simulink model "BlinkerCAN"  (R2017b)
settings: Solver=FixedStepAuto  StartTime=0.0  StopTime=10.0  RelTol=1e-3
PreLoadFcn:
  | waijung.modelPreload; % Required for working with Waijung Blockset. Do not remove.
undefined symbols (not defined in the file): HSEOSC, Link, LQFP100, ST, STM32F407VG
libraries: simulink x22, hdlsllib x17, stm32f4_canbus_lib x5, stm32f4_io_lib x1, stm32f4_device_config_lib x1
CloseFcn:
  | waijung.modelClose; % Required for working with Waijung Blockset. Do not remove.
settings Model: Creator=labuser  LastModifiedBy=labuser
settings OptimizationCC: DefaultParameterBehavior=Inlined  PassReuseOutputArgsAs=Individual arguments
settings DebuggingCC: ParameterTunabilityLossMsg=error
settings HardwareCC: ProdBitPerPointer=32  ProdBitPerSizeT=32  ProdBitPerPtrDiffT=32  ProdLargestAtomicFloat=None  ProdIntDivRoundTo=Undefined  ProdWordSize=32  ProdHWDeviceType=ARM Compatible->Cortex - M4  TargetEndianess=LittleEndian  TargetHWDeviceType=ARM Compatible->Cortex - M4
settings SFSimCC: MATLABDynamicMemAlloc=off
settings RTWCC: SystemTargetFile=stm32f4.tlc  GenerateMakefile=off  TemplateMakefile=ert_default_tmf  Description=STM32F4 Target  GenerateReport=on  IncludeHyperlinkInReport=on  LaunchReport=on  GenerateTraceInfo=on  GenerateTraceReport=on  GenerateTraceReportSl=on  GenerateTraceReportSf=on  GenerateTraceReportEml=on
settings CodeAppCC: ForceParamTrailComments=on  IgnoreCustomStorageClasses=off  OperatorAnnotations=on  SimulinkDataObjDesc=on  SFDataObjDesc=on  InsertBlockDesc=on
settings STFCustomTargetCC: TargetLangStandard=C99 (ISO)  MultiwordLength=256  ModelReferenceCompliant=off  CombineOutputUpdateFcns=on  ERTCustomFileBanners=on  SupportContinuousTime=off  SupportNonInlinedSFcns=off  RemoveResetFunc=on  MATLABClassNameForMDSCustomization=Simulink.SoftwareTarget.ERTCustomization  GRTInterface=off  SystemTargetFile=stm32f4.tlc
settings ERTTargetCC: TargetLangStandard=C99 (ISO)  ModelReferenceCompliant=off  ParMdlRefBuildCompliant=off  CompOptLevelCompliant=off  ConcurrentExecutionCompliant=off  ModelStepFunctionPrototypeControlCompliant=off  CPPClassGenCompliant=off  UseToolchainInfoCompliant=off  InlinedParameterPlacement=NonHierarchical  ERTSrcFileBannerTemplate=stm32f4_code_template.cgt  ERTHdrFileBannerTemplate=stm32f4_code_template.cgt  ERTDataSrcFileTemplate=stm32f4_code_template.cgt  ERTDataHdrFileTemplate=stm32f4_code_template.cgt  ERTCustomFileTemplate=stm32f4_file_process.tlc

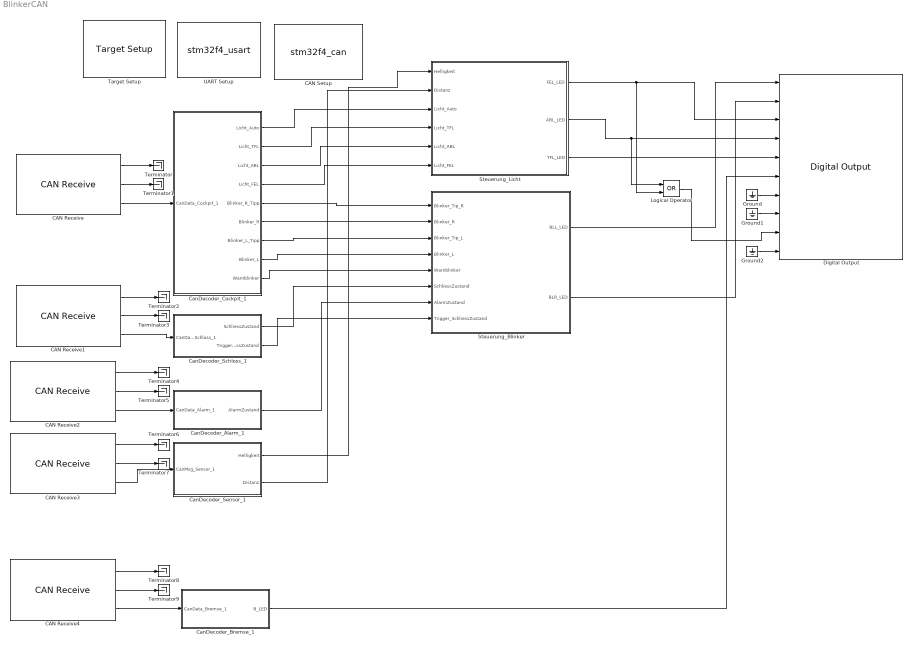
== system BlinkerCAN ==
  CAN Receive : stm32f4_canbus_lib/CAN Receive  conf=Rx  canmodule=1  idtype=Standard  filtertype=Specific  id=14  idmask=00000000  enableisr=off  usedlc=off  datatype=single  data0type=uint8  data1type=Not used  data2type=Not used  data3type=Not used  data4type=Not used  data5type=Not used  data6type=Not used  data7type=Not used  buffersize=8  sampletime=-1  sampletimestr=-1  blockid=CANReceive  inputarray=[]  inputlabelarray={}  outputarray=[ 5, 7, 3]  outputlabelarray={ 'Msg Pending','ID', 'D0 (uint8)' }  compat=0  confstr="[\"Standard\",\"Specific\",\"14\",\"0\",\"off\",\"uint8\",\"Not used\",\"Not used\",\"Not used\",\"Not used\",\"Not used\",\"Not used\",\"Not used\",\"8\",\"1C0\",\"0\",\"FFE0\",\"4\"]"
  CAN Receive1 : stm32f4_canbus_lib/CAN Receive  conf=Rx  canmodule=1  idtype=Standard  filtertype=Specific  id=25  idmask=00000000  enableisr=off  usedlc=off  datatype=single  data0type=uint8  data1type=Not used  data2type=Not used  data3type=Not used  data4type=Not used  data5type=Not used  data6type=Not used  data7type=Not used  buffersize=8  sampletime=-1  sampletimestr=-1  blockid=CANReceive1  inputarray=[]  inputlabelarray={}  outputarray=[ 5, 7, 3]  outputlabelarray={ 'Msg Pending','ID', 'D0 (uint8)' }  compat=0  confstr="[\"Standard\",\"Specific\",\"25\",\"0\",\"off\",\"uint8\",\"Not used\",\"Not used\",\"Not used\",\"Not used\",\"Not used\",\"Not used\",\"Not used\",\"8\",\"320\",\"0\",\"FFE0\",\"4\"]"
  CAN Receive2 : stm32f4_canbus_lib/CAN Receive  conf=Rx  canmodule=1  idtype=Standard  filtertype=Specific  id=24  idmask=00000000  enableisr=off  usedlc=off  datatype=single  data0type=uint8  data1type=Not used  data2type=Not used  data3type=Not used  data4type=Not used  data5type=Not used  data6type=Not used  data7type=Not used  buffersize=8  sampletime=-1  sampletimestr=-1  blockid=CANReceive2  inputarray=[]  inputlabelarray={}  outputarray=[ 5, 7, 3]  outputlabelarray={ 'Msg Pending','ID', 'D0 (uint8)' }  compat=0  confstr="[\"Standard\",\"Specific\",\"24\",\"0\",\"off\",\"uint8\",\"Not used\",\"Not used\",\"Not used\",\"Not used\",\"Not used\",\"Not used\",\"Not used\",\"8\",\"300\",\"0\",\"FFE0\",\"4\"]"
  CAN Receive3 : stm32f4_canbus_lib/CAN Receive  conf=Rx  canmodule=1  idtype=Standard  filtertype=Specific  id=32  idmask=00000000  enableisr=off  usedlc=off  datatype=single  data0type=uint16  data1type=Not used  data2type=Not used  data3type=Not used  data4type=Not used  data5type=Not used  data6type=Not used  data7type=Not used  buffersize=8  sampletime=-1  sampletimestr=-1  blockid=CANReceive3  inputarray=[]  inputlabelarray={}  outputarray=[ 5, 7, 5]  outputlabelarray={ 'Msg Pending','ID', 'D0 (uint16)' }  compat=0  confstr="[\"Standard\",\"Specific\",\"32\",\"0\",\"off\",\"uint16\",\"Not used\",\"Not used\",\"Not used\",\"Not used\",\"Not used\",\"Not used\",\"Not used\",\"8\",\"400\",\"0\",\"FFE0\",\"4\"]"
  CAN Receive4 : stm32f4_canbus_lib/CAN Receive  conf=Rx  canmodule=1  idtype=Standard  filtertype=Specific  id=10  idmask=00000000  enableisr=off  usedlc=off  datatype=single  data0type=uint8  data1type=Not used  data2type=Not used  data3type=Not used  data4type=Not used  data5type=Not used  data6type=Not used  data7type=Not used  buffersize=8  sampletime=-1  sampletimestr=-1  blockid=CANReceive4  inputarray=[]  inputlabelarray={}  outputarray=[ 5, 7, 3]  outputlabelarray={ 'Msg Pending','ID', 'D0 (uint8)' }  compat=0  confstr="[\"Standard\",\"Specific\",\"10\",\"0\",\"off\",\"uint8\",\"Not used\",\"Not used\",\"Not used\",\"Not used\",\"Not used\",\"Not used\",\"Not used\",\"8\",\"140\",\"0\",\"FFE0\",\"4\"]"
  CAN Setup : S-Function  FunctionName=stm32f4_can  Parameters=conf,canmodule,0,inputarray,outputarray,'','',confstr,sampletime,sampletimestr,blockid  SFunctionDeploymentMode=off  EnableBusSupport=off  mask(stm32f4_can){conf=Setup, canmodule=1, advance=off, bitrate_select=125000, sjw=1tq, bs1=14tq, bs2=6tq, timingconf=Prescaler, brp=16, bitrate=125000, tq=3.8095e-07, autoretransmission=Disable, remaptxpin=D1, remaprxpin=D0, sampletime=-1, sampletimestr=-1, blockid=CANSetup, inputarray=[], inputlabelarray={}, outputarray=[], outputlabelarray={}, compat=0, confstr=["125000","16","D","1","D","0","1tq","14tq","6tq","ENABLE"], presc=16, txportstr=D, txpinstr=1, rxportstr=D, rxpinstr=0, lastmodule=1}
      mask prompts: conf "Configuration"; canmodule "CAN Module"; advance "Advance configuration"; bitrate_select "Baud rate (bps)"; sjw "Resync Jump Width (SJW)"; bs1 "Bit segment 1 (BS1) + PROP_SEG"; bs2 "Bit segment 2 (BS2)"; timingconf "Adjust"; brp "Baud rate prescaler (BRP)"; bitrate "Baud rate (bps)"; tq "Time Quantum (Second), tq"; autoretransmission "Auto Re-transmission"; remaptxpin "CAN Tx pin"; remaprxpin "CAN Rx pin"; sampletime "Sample time (sec)"; sampletimestr "Compiled sample time (sec) in string"; inputarray "Input port"; inputlabelarray "Input port label"; outputarray "Output port"; outputlabelarray "Output port label"; compat "Compatibility (Reserved for future use)"; confstr "Configuration String"; presc "Prescale"; txportstr "Tx port string"; txpinstr "Tx pin string"; rxportstr "Rx port string"; rxpinstr "Rx pin string"; lastmodule "Last module selected"
      mask help:
      | This block setups CAN Module.
      |
      | Auto Re-transmission,
      |  - Enable: The CAN hardware will automatically retransmit the message until it has been
      | successfully transmitted according to the CAN standard.
      |  - Disable: A message will be transmitted only once, independently of the transmission result
      | (successful, error or arbitration lost).
      mask init:
      | stm32f4_can_callback('init');
      mask Help: web(fullfile(waijungdocroot,'stm32f4_can_setup.htm'), '-browser')
      mask TypeOptions conf: Setup
      mask TypeOptions canmodule: 1 | 2
      mask Callback canmodule: stm32f4_can_callback('canmodule');
      mask Callback advance: stm32f4_can_callback('advance');
      mask TypeOptions bitrate_select: 125000 | 250000 | 500000 | 1000000
      mask Callback bitrate_select: stm32f4_can_callback('bitrate_select');
      mask TypeOptions sjw: 1tq | 2tq | 3tq | 4tq
      mask TypeOptions bs1: 1tq | 2tq | 3tq | 4tq | 5tq | 6tq | 7tq | 8tq | 9tq | 10tq | 11tq | 12tq | 13tq | 14tq | 15tq | 16tq
      mask Callback bs1: stm32f4_can_callback('timingconf');
      mask TypeOptions bs2: 1tq | 2tq | 3tq | 4tq | 5tq | 6tq | 7tq | 8tq
      mask Callback bs2: stm32f4_can_callback('timingconf');
      mask TypeOptions timingconf: Prescaler | Baudrate
      mask Callback timingconf: stm32f4_can_callback('timingconf');
      mask Callback brp: stm32f4_can_callback('timingconf');
      mask Callback bitrate: stm32f4_can_callback('timingconf');
      mask TypeOptions autoretransmission: Enable | Disable
      mask TypeOptions remaptxpin: Not used | A12 | B9 | D1
      mask Callback remaptxpin: stm32f4_can_callback('remaptxpin');
      mask TypeOptions remaprxpin: Not used | A11 | B8 | D0
      mask Callback remaprxpin: stm32f4_can_callback('remaprxpin');
      mask Callback sampletime: stm32f4_can_callback('sampletime');
      mask Callback sampletimestr: stm32f4_can_callback('sampletimestr');
      mask Callback blockid: stm32f4_can_callback('blockid');
      mask Display: text(0.5, 0.5, 'CAN1_Setup\nSpeed (bps): 125000\nTx/Rx pin: D1/D0','ver','middle','hor','center');
  CanDecoder_Alarm_1 : Subsystem
  CanDecoder_Bremse_1 : Subsystem
  CanDecoder_Cockpit_1 : Subsystem
  CanDecoder_Schloss_1 : Subsystem
  CanDecoder_Sensor_1 : Subsystem
  Digital Output : stm32f4_io_lib/Digital Output  use_bitband=on  port=C  speed=100  porttype=Push Pull  porttypestr=PP  use_pin0=on  use_pin1=on  use_pin2=on  use_pin3=on  use_pin4=on  use_pin5=on  use_pin6=on  use_pin7=on  use_pin8=on  use_pin9=on  use_pin10=off  use_pin11=off  use_pin12=off  use_pin13=off  use_pin14=off  use_pin15=off  pinstr=GPIO_Pin_0 | GPIO_Pin_1 | GPIO_Pin_2 | GPIO_Pin_3 | GPIO_Pin_4 | GPIO_Pin_5 | GPIO_Pin_6 | GPIO_Pin_7 | GPIO_Pin_8 | GPIO_Pin_9  usedpinarray="[1  1  1  1  1  1  1  1  1  1  0  0  0  0  0  0]"  bitbandingstr=|  sampletime=-1  sampletimestr=-1  blockid=DigitalOutput  enablecustomportlabel=off  globalinit=off  cinputportlabel=In1, In2  coutputportlabel=0
      | #define DigitalOutput_C0 Peripheral_BB(GPIOC->ODR, 0)  /* Output pin */
      | #define DigitalOutput_C1 Peripheral_BB(GPIOC->ODR, 1)  /* Output pin */
      | #define DigitalOutput_C2 Peripheral_BB(GPIOC->ODR, 2)  /* Output pin */
      | #define DigitalOutput_C3 Peripheral_BB(GPIOC->ODR, 3)  /* Output pin */
      | #define DigitalOutput_C4 Peripheral_BB(GPIOC->ODR, 4)  /* Output pin */
      | #define DigitalOutput_C5 Peripheral_BB(GPIOC->ODR, 5)  /* Output pin */
      | #define DigitalOutput_C6 Peripheral_BB(GPIOC->ODR, 6)  /* Output pin */
      | #define DigitalOutput_C7 Peripheral_BB(GPIOC->ODR, 7)  /* Output pin */
      | #define DigitalOutput_C8 Peripheral_BB(GPIOC->ODR, 8)  /* Output pin */
      | #define DigitalOutput_C9 Peripheral_BB(GPIOC->ODR, 9)  /* Output pin */
      settings: SourceProductName=Waijung Blockset
  Ground : Ground
  Ground1 : Ground
  Ground2 : Ground
  Logical Operator : Logic  Operator=OR  AllPortsSameDT=off  OutDataTypeStr=boolean
  Steuerung_Blinker : Stateflow chart  TreatAsAtomicUnit=on
  Steuerung_Licht : Stateflow chart  TreatAsAtomicUnit=on
  Target Setup : stm32f4_device_config_lib/Target Setup  Priority=100  compiler=GNU ARM  previous_compiler=GNU ARM  mcu=STM32F407VG (LQFP100)  mcustr=STM32F407VG  clockconfig=HSEOSC-8MHz  system_stm32f4xx_c_path=C:\Users\labuser\Desktop\waijung17_03a\targets\stm32f4_target\stm32f4\utils\system_stm32f4xx_default\STM32F40_41xxx\hseosc8mhz  showmemoryconfiguration=off  stacksize=0x2000  heapsize=0x2000  enableautocompiledownload=on  fullchiperase=off  programmerinterface=ST-Link  editctrlstr=on  compilercontrolstr=$(patsubst %, -I%, .) -mcpu=cortex-m4 -mthumb -mthumb-interwork -mfloat-abi=hard -mfpu=fpv4-sp-d16 -ffast-math -Wall -Wextra -Ofast  assemblercontrolstr=$(patsubst %, -I%, .) -mcpu=cortex-m4 -mthumb -mthumb-interwork -mfloat-abi=hard -mfpu=fpv4-sp-d16 -ffast-math -Wall -Wextra -Ofast -Wa,-amhls=$(<:.s=.lst) -D__STACK_SIZE=$(STACK_SIZE) -D__HEAP_SIZE=$(HEAP_SIZE)  linkercontrolstr=-T$(LD_SCRIPT) -g -Wl,-Map=$(MAP),--cref,--no-warn-mismatch -mcpu=cortex-m4 -mthumb -mthumb-interwork -mfloat-abi=hard -mfpu=fpv4-sp-d16 -specs=nosys.specs  runafterdownload=on  execprofile=None  profileruart=3  profilerbaud=500000  profilertxpin=D8  profilerinitstr=0.01,168000000,1680000,500000,0  manualsetsampletime=off  sampletime=0.01  blockid=TargetSetup  systickreloadvalue=1680000  hseval=8000000  lastprofileruart=3  hclk=168000000  flashorigin=0x8000000  flashlength=1024k  ramorigin=0x20000000  ramlength=128k  useextram=off
      settings: SourceProductName=Waijung Blockset
  Terminator{,1..9} (10 alike) : Terminator
  UART Setup : S-Function  Priority=1  FunctionName=stm32f4_usart  Parameters=configuration,uartmodule,transfer,baudrate,inputtype,outputtype,confstr,binheaderarray,binterminatorarray,asciiheader,asciiterminator,bindatalength,packetmode,varname,sampletime,sampletimestr,blockid  SFunctionDeploymentMode=off  EnableBusSupport=off  mask(stm32f4_usart){configuration=Setup, uartmodule=2, baudrate=115200, databits=8, parity=No, stopbit=1, remaptxpin=A2, remaprxpin=A3, flowcontrol=None, remapctspin=Not used, remaprtspin=Not used, advanceoptions=off, rxbuffersize=512, txbuffersize=512, transfer=Blocking, packetmode=Ascii, binheader='7E 7E', binterminator='03 03', porttype_double=1, porttype_single=0, porttype_int8=1, porttype_uint8=0, porttype_int16=0, porttype_uint16=0, porttype_int32=0, porttype_uint32=0, asciiformat='%d,%f', rx_asciiterminator=CRLF (0x0D 0x0A - "\r\n"), tx_asciiterminator=CR (0x0D - "\r"), storagename=<empty>, varname=, inputtype=[0], outputtype=[0], binheaderarray=[0], binterminatorarray=[0], bindatalength=0, asciiheader='', asciiterminator=[0], sampletime=-1, sampletimestr=-1, blockid=UARTSetup, confstr=[ "dummy", "1", "A", "2", "1", "A", "3", "0", "*", "*", "0", "*", "*", "1", "4", "6", "1", "4", "5", "512", "512", "1", "2", "115200", "8", "No", "1", "None", "USART2"], lastmodule=2}
      mask prompts: uartmodule "UART Module"; baudrate "Baud rate (bps)"; databits "Data bits"; stopbit "Stop bit"; remaptxpin "Tx Pin"; remaprxpin "Rx Pin"; flowcontrol "Hardware flow control"; remapctspin "HW Flow control, CTS Pin"; remaprtspin "HW Flow control, RTS Pin"; advanceoptions "Advance options"; rxbuffersize "Rx buffer size (bytes)"; txbuffersize "Tx buffer size (bytes)"; packetmode "Packet mode"; binheader "Binary header (example: '7E 7E')"; binterminator "Binary terminator (example: '03 03')"; porttype_double "Number of data port, type DOUBLE"; porttype_single "Number of data port, type SINGLE"; porttype_int8 "Number of data port, type INT8"; porttype_uint8 "Number of data port, type UINT8"; porttype_int16 "Number of data port, type INT16"; porttype_uint16 "Number of data port, type UINT16"; porttype_int32 "Number of data port, type INT32"; porttype_uint32 "Number of data port, type UINT32"; asciiformat "Ascii format"; rx_asciiterminator "End of packet"; tx_asciiterminator "End of packet"; storagename "Buffer"; varname "Var name"; inputtype "Input data type"; outputtype "Output data type"; binheaderarray "Binary header"; binterminatorarray "Binary terminator"; bindatalength "Binary data length"; asciiheader "Ascii header (printf format)"; asciiterminator "Ascii terminator"; sampletime "Sample time (sec)"; sampletimestr "Compiled sample time (sec) in string"; confstr "Configuration string"; lastmodule "Last module selected"
      mask help:
      | Default STM32F4DISCOVERY + aMG F4 Connect 2 + aMG USB Converter N2 settings use
      |
      | USART3, Tx D8, Rx D9 and USB Serial Converter A.
      mask init:
      | stm32f4_usart_callback('init');
      mask Help: web(fullfile(waijungdocroot,'stm32f4_usart_setup.htm'), '-browser')
      mask TypeOptions configuration: Setup | Tx | Rx
      mask Callback configuration: stm32f4_usart_callback('configuration');
      mask TypeOptions uartmodule: 1 | 2 | 3 | 4 | 5 | 6
      mask Callback uartmodule: stm32f4_usart_callback('uartmodule');
      mask Callback baudrate: stm32f4_usart_callback('baudrate');
      mask TypeOptions databits: 8
      mask TypeOptions parity: No | Odd | Even
      mask TypeOptions stopbit: 0.5 | 1 | 1.5 | 2
      mask TypeOptions remaptxpin: Not used | A2 | D5
      mask TypeOptions remaprxpin: Not used | A3 | D6
      mask TypeOptions flowcontrol: None | RTS | CTS | RTS/CTS
      mask Callback flowcontrol: stm32f4_usart_callback('flowcontrol');
      mask TypeOptions remapctspin: Not used | A0 | D3
      mask TypeOptions remaprtspin: Not used | A1 | D4
      mask Callback advanceoptions: stm32f4_usart_callback('advanceoptions');
      mask TypeOptions rxbuffersize: 16 | 32 | 64 | 128 | 256 | 512 | 1024 | 2048
      mask TypeOptions txbuffersize: 16 | 32 | 64 | 128 | 256 | 512 | 1024 | 2048
      mask TypeOptions transfer: Blocking | Non-Blocking
      mask Callback transfer: stm32f4_usart_callback('transfer');
      mask TypeOptions packetmode: Ascii | Binary | String Buffer
      mask Callback packetmode: stm32f4_usart_callback('packetmode');
      mask Callback binheader: stm32f4_usart_callback('binheader');
      mask Callback binterminator: stm32f4_usart_callback('binterminator');
      mask Callback porttype_double: stm32f4_usart_callback('porttype');
      mask Callback porttype_single: stm32f4_usart_callback('porttype');
      mask Callback porttype_int8: stm32f4_usart_callback('porttype');
      mask Callback porttype_uint8: stm32f4_usart_callback('porttype');
      mask Callback porttype_int16: stm32f4_usart_callback('porttype');
      mask Callback porttype_uint16: stm32f4_usart_callback('porttype');
      mask Callback porttype_int32: stm32f4_usart_callback('porttype');
      mask Callback porttype_uint32: stm32f4_usart_callback('porttype');
      mask Callback asciiformat: stm32f4_usart_callback('asciiformat');
      mask TypeOptions rx_asciiterminator: CR (0x0D - "\r") | LF (0x0A - "\n") | CRLF (0x0D 0x0A - "\r\n")
      mask Callback rx_asciiterminator: stm32f4_usart_callback('rx_asciiterminator');
      mask TypeOptions tx_asciiterminator: CR (0x0D - "\r") | LF (0x0A - "\n") | CRLF (0x0D 0x0A - "\r\n") | None
      mask Callback tx_asciiterminator: stm32f4_usart_callback('tx_asciiterminator');
      mask TypeOptions storagename: <empty>
      mask Callback storagename: stm32f4_usart_callback('storagename');
      mask Callback varname: stm32f4_usart_callback('varname');
      mask Callback sampletime: stm32f4_usart_callback('sampletime');
      mask Callback sampletimestr: stm32f4_usart_callback('sampletimestr');
      mask Callback blockid: stm32f4_usart_callback('blockid');
      mask Display: text(0.5, 0.5, 'Module: USART2_Setup\nBaud (Bps): 115200\nDMA Buffer: 512/512\nTx/Rx Pin: A2/A3','ver','middle','hor','center');
  wires:
  Steuerung_Blinker/1(BLL_LED) -> Digital Output/1
  Steuerung_Licht/3(TFL_LED) -> Digital Output/5
  Steuerung_Blinker/2(BLR_LED) -> Digital Output/2
  Steuerung_Licht/1(FEL_LED) -> Logical Operator/2, Digital Output/3
  Steuerung_Licht/2(ABL_LED) -> Logical Operator/1, Digital Output/4
  CAN Receive1/3 -> CanDecoder_Schloss_1/1(CanData_Schloss_1)
  CAN Receive2/3 -> CanDecoder_Alarm_1/1(CanData_Alarm_1)
  CanDecoder_Schloss_1/1(SchliessZustand) -> Steuerung_Blinker/6(SchliessZustand)
  CanDecoder_Alarm_1/1(AlarmZustand) -> Steuerung_Blinker/7(AlarmZustand)
  CanDecoder_Cockpit_1/9(Warnblinker) -> Steuerung_Blinker/5(Warnblinker)
  CanDecoder_Cockpit_1/8(Blinker_L) -> Steuerung_Blinker/4(Blinker_L)
  CanDecoder_Cockpit_1/7(Blinker_L_Tipp) -> Steuerung_Blinker/3(Blinker_Tip_L)
  CanDecoder_Cockpit_1/6(Blinker_R) -> Steuerung_Blinker/2(Blinker_R)
  CanDecoder_Cockpit_1/5(Blinker_R_Tipp) -> Steuerung_Blinker/1(Blinker_Tip_R)
  CanDecoder_Cockpit_1/4(Licht_FEL) -> Steuerung_Licht/6(Licht_FEL)
  CanDecoder_Cockpit_1/3(Licht_ABL) -> Steuerung_Licht/5(Licht_ABL)
  CanDecoder_Cockpit_1/2(Licht_TFL) -> Steuerung_Licht/4(Licht_TFL)
  CanDecoder_Cockpit_1/1(Licht_Auto) -> Steuerung_Licht/3(Licht_Auto)
  CAN Receive/1 -> Terminator/1
  CAN Receive1/1 -> Terminator2/1
  CAN Receive1/2 -> Terminator3/1
  CAN Receive2/1 -> Terminator4/1
  CAN Receive2/2 -> Terminator5/1
  CAN Receive3/1 -> Terminator6/1
  CAN Receive3/3 -> CanDecoder_Sensor_1/1(CanMsg_Sensor_1)
  CAN Receive3/2 -> Terminator7/1
  CAN Receive/3 -> CanDecoder_Cockpit_1/1(CanData_Cockpit_1)
  CanDecoder_Sensor_1/1(Helligkeit) -> Steuerung_Licht/1(Helligkeit)
  CanDecoder_Sensor_1/2(Distanz) -> Steuerung_Licht/2(Distanz)
  CAN Receive4/1 -> Terminator8/1
  CAN Receive4/2 -> Terminator9/1
  CAN Receive4/3 -> CanDecoder_Bremse_1/1(CanData_Bremse_1)
  CanDecoder_Bremse_1/1(B_LED) -> Digital Output/6
  Logical Operator/1 -> Digital Output/9
  CanDecoder_Schloss_1/2(Trigger_SchliessZustand) -> Steuerung_Blinker/8(Trigger_SchliessZustand)
  CAN Receive/2 -> Terminator1/1
  Ground1/1 -> Digital Output/8
  Ground2/1 -> Digital Output/10
  Ground/1 -> Digital Output/7

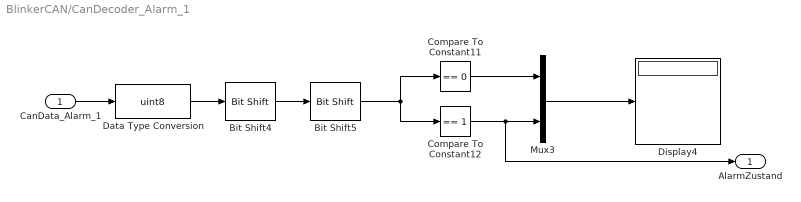
== system BlinkerCAN/CanDecoder_Alarm_1 ==
  CanData_Alarm_1 : Inport
  Bit Shift4 : hdlsllib/Logic and Bit Operations/Bit Shift  mode=Shift Left Logical  N=7
      settings: SourceProductName=HDL Coder  SourceProductBaseCode=HD
  Bit Shift5 : hdlsllib/Logic and Bit Operations/Bit Shift  mode=Shift Right Logical  N=7
      settings: SourceProductName=HDL Coder  SourceProductBaseCode=HD
  Compare To Constant11 : simulink/Logic and Bit Operations/Compare To Constant  relop===  const=0  OutDataTypeStr=boolean
  Compare To Constant12 : simulink/Logic and Bit Operations/Compare To Constant  relop===  const=1  OutDataTypeStr=boolean
  Data Type Conversion : DataTypeConversion  OutDataTypeStr=uint8
  Display4 : Display
  Mux3 : Mux  Inputs=2
  AlarmZustand : Outport
  wires:
  CanData_Alarm_1/1 -> Data Type Conversion/1
  Compare To Constant12/1 -> AlarmZustand/1, Mux3/2
  Bit Shift4/1 -> Bit Shift5/1
  Compare To Constant11/1 -> Mux3/1
  Bit Shift5/1 -> Compare To Constant11/1, Compare To Constant12/1
  Mux3/1 -> Display4/1
  Data Type Conversion/1 -> Bit Shift4/1

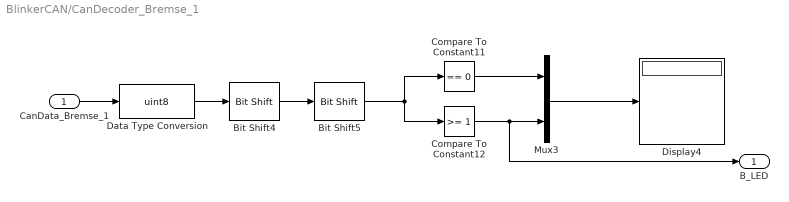
== system BlinkerCAN/CanDecoder_Bremse_1 ==
  CanData_Bremse_1 : Inport
  Bit Shift4 : hdlsllib/Logic and Bit Operations/Bit Shift  mode=Shift Left Logical  N=5
      settings: SourceProductName=HDL Coder  SourceProductBaseCode=HD
  Bit Shift5 : hdlsllib/Logic and Bit Operations/Bit Shift  mode=Shift Right Logical  N=5
      settings: SourceProductName=HDL Coder  SourceProductBaseCode=HD
  Compare To Constant11 : simulink/Logic and Bit Operations/Compare To Constant  relop===  const=0  OutDataTypeStr=boolean
  Compare To Constant12 : simulink/Logic and Bit Operations/Compare To Constant  relop=>=  const=1  OutDataTypeStr=boolean
  Data Type Conversion : DataTypeConversion  OutDataTypeStr=uint8
  Display4 : Display
  Mux3 : Mux  Inputs=2
  B_LED : Outport
  wires:
  Data Type Conversion/1 -> Bit Shift4/1
  Mux3/1 -> Display4/1
  Bit Shift5/1 -> Compare To Constant12/1, Compare To Constant11/1
  Compare To Constant11/1 -> Mux3/1
  Bit Shift4/1 -> Bit Shift5/1
  Compare To Constant12/1 -> Mux3/2, B_LED/1
  CanData_Bremse_1/1 -> Data Type Conversion/1

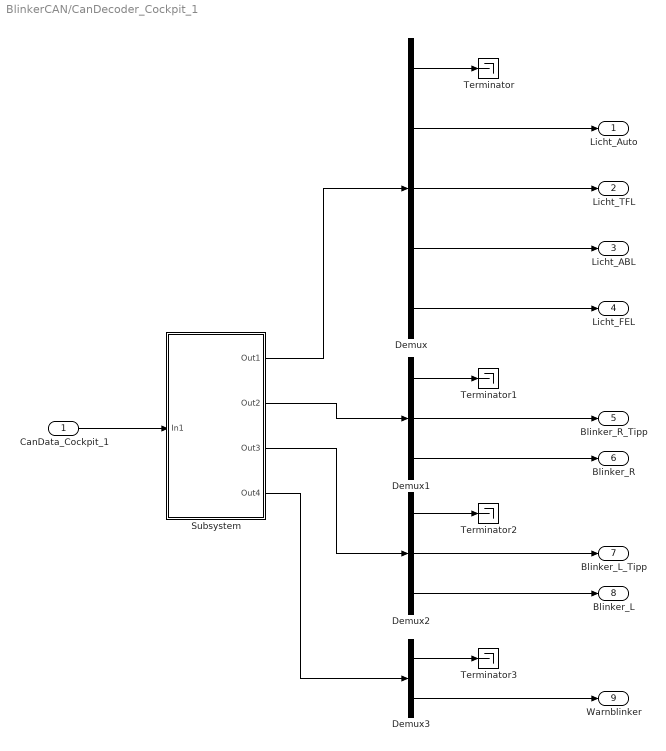
== system BlinkerCAN/CanDecoder_Cockpit_1 ==
  CanData_Cockpit_1 : Inport
  Demux : Demux  Outputs=5
  Demux1 : Demux  Outputs=3
  Demux2 : Demux  Outputs=3
  Demux3 : Demux  Outputs=2
  Subsystem : Subsystem
  Terminator{,1..3} (4 alike) : Terminator
  Licht_Auto : Outport
  Licht_TFL : Outport  Port=2
  Licht_ABL : Outport  Port=3
  Licht_FEL : Outport  Port=4
  Blinker_R_Tipp : Outport  Port=5
  Blinker_R : Outport  Port=6
  Blinker_L_Tipp : Outport  Port=7
  Blinker_L : Outport  Port=8
  Warnblinker : Outport  Port=9
  wires:
  CanData_Cockpit_1/1 -> Subsystem/1(In1)
  Subsystem/1(Out1) -> Demux/1
  Demux/1 -> Terminator/1
  Demux/2 -> Licht_Auto/1
  Demux/3 -> Licht_TFL/1
  Demux/4 -> Licht_ABL/1
  Demux/5 -> Licht_FEL/1
  Demux1/1 -> Terminator1/1
  Demux1/3 -> Blinker_R/1
  Demux1/2 -> Blinker_R_Tipp/1
  Demux2/1 -> Terminator2/1
  Demux2/2 -> Blinker_L_Tipp/1
  Demux2/3 -> Blinker_L/1
  Subsystem/2(Out2) -> Demux1/1
  Subsystem/3(Out3) -> Demux2/1
  Demux3/2 -> Warnblinker/1
  Demux3/1 -> Terminator3/1
  Subsystem/4(Out4) -> Demux3/1

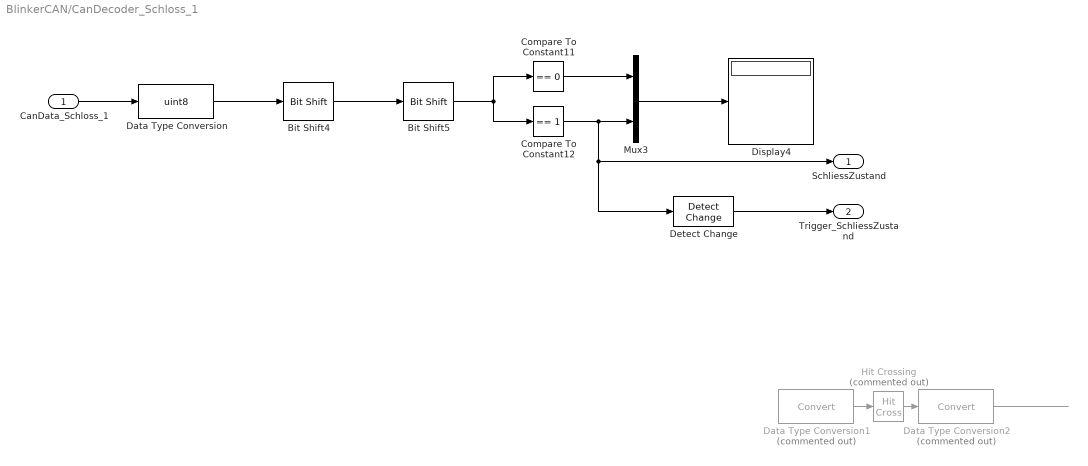
== system BlinkerCAN/CanDecoder_Schloss_1 ==
  CanData_Schloss_1 : Inport
  Bit Shift4 : hdlsllib/Logic and Bit Operations/Bit Shift  mode=Shift Left Logical  N=7
      settings: SourceProductName=HDL Coder  SourceProductBaseCode=HD
  Bit Shift5 : hdlsllib/Logic and Bit Operations/Bit Shift  mode=Shift Right Logical  N=7
      settings: SourceProductName=HDL Coder  SourceProductBaseCode=HD
  Compare To Constant11 : simulink/Logic and Bit Operations/Compare To Constant  relop===  const=0  OutDataTypeStr=boolean
  Compare To Constant12 : simulink/Logic and Bit Operations/Compare To Constant  relop===  const=1  OutDataTypeStr=boolean
  Data Type Conversion : DataTypeConversion  OutDataTypeStr=uint8
  Data Type Conversion1 : DataTypeConversion  Commented=on
  Data Type Conversion2 : DataTypeConversion  Commented=on
  Detect Change : simulink/Logic and Bit Operations/Detect Change  vinit=0  OutDataTypeStr=boolean
  Display4 : Display
  Hit Crossing : HitCross  Commented=on  HitCrossingOffset=0.5
  Mux3 : Mux  Inputs=2
  SchliessZustand : Outport
  Trigger_SchliessZustand : Outport  Port=2
  wires:
  Mux3/1 -> Display4/1
  Compare To Constant11/1 -> Mux3/1
  Compare To Constant12/1 -> Detect Change/1, SchliessZustand/1, Mux3/2
  Bit Shift4/1 -> Bit Shift5/1
  Bit Shift5/1 -> Compare To Constant11/1, Compare To Constant12/1
  Data Type Conversion/1 -> Bit Shift4/1
  CanData_Schloss_1/1 -> Data Type Conversion/1
  Data Type Conversion1/1 -> Hit Crossing/1
  Data Type Conversion2/1 -> ?
  Hit Crossing/1 -> Data Type Conversion2/1
  Detect Change/1 -> Trigger_SchliessZustand/1

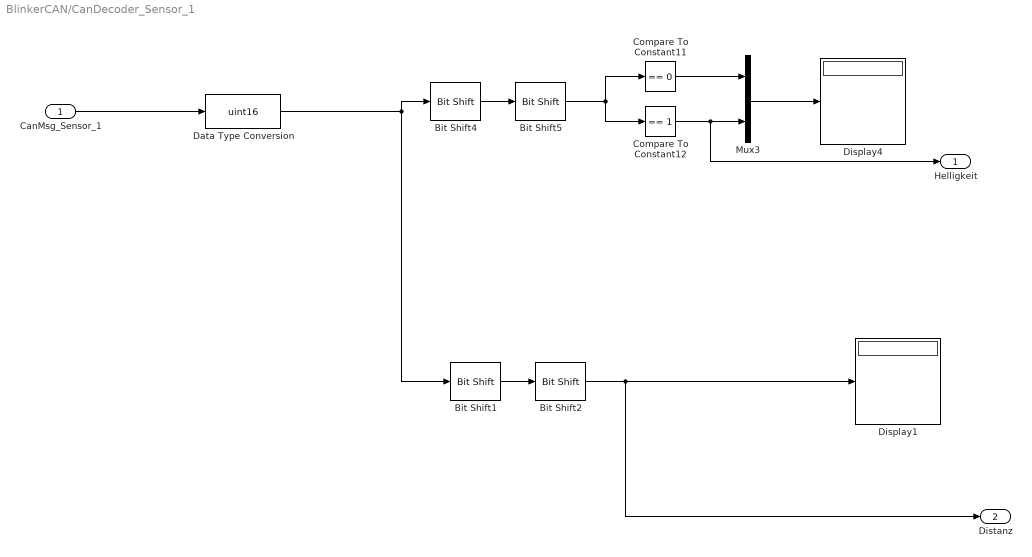
== system BlinkerCAN/CanDecoder_Sensor_1 ==
  CanMsg_Sensor_1 : Inport
  Bit Shift1 : hdlsllib/Logic and Bit Operations/Bit Shift  mode=Shift Left Logical  N=6
      settings: SourceProductName=HDL Coder  SourceProductBaseCode=HD
  Bit Shift2 : hdlsllib/Logic and Bit Operations/Bit Shift  mode=Shift Right Logical  N=7
      settings: SourceProductName=HDL Coder  SourceProductBaseCode=HD
  Bit Shift4 : hdlsllib/Logic and Bit Operations/Bit Shift  mode=Shift Left Logical  N=15
      settings: SourceProductName=HDL Coder  SourceProductBaseCode=HD
  Bit Shift5 : hdlsllib/Logic and Bit Operations/Bit Shift  mode=Shift Right Logical  N=15
      settings: SourceProductName=HDL Coder  SourceProductBaseCode=HD
  Compare To Constant11 : simulink/Logic and Bit Operations/Compare To Constant  relop===  const=0  OutDataTypeStr=boolean
  Compare To Constant12 : simulink/Logic and Bit Operations/Compare To Constant  relop===  const=1  OutDataTypeStr=boolean
  Data Type Conversion : DataTypeConversion  OutDataTypeStr=uint16
  Display1 : Display
  Display4 : Display
  Mux3 : Mux  Inputs=2
  Helligkeit : Outport
  Distanz : Outport  Port=2
  wires:
  CanMsg_Sensor_1/1 -> Data Type Conversion/1
  Compare To Constant12/1 -> Helligkeit/1, Mux3/2
  Bit Shift4/1 -> Bit Shift5/1
  Compare To Constant11/1 -> Mux3/1
  Bit Shift5/1 -> Compare To Constant11/1, Compare To Constant12/1
  Mux3/1 -> Display4/1
  Bit Shift2/1 -> Distanz/1, Display1/1
  Bit Shift1/1 -> Bit Shift2/1
  Data Type Conversion/1 -> Bit Shift1/1, Bit Shift4/1

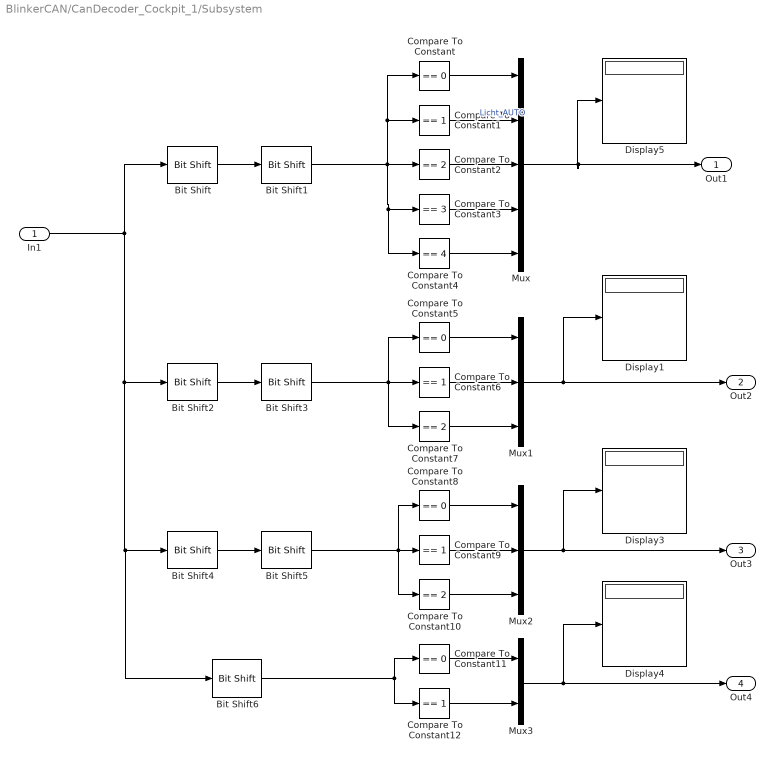
== system BlinkerCAN/CanDecoder_Cockpit_1/Subsystem ==
  In1 : Inport
  Bit Shift : hdlsllib/Logic and Bit Operations/Bit Shift  mode=Shift Left Logical  N=5
      settings: SourceProductName=HDL Coder  SourceProductBaseCode=HD
  Bit Shift1 : hdlsllib/Logic and Bit Operations/Bit Shift  mode=Shift Right Logical  N=5
      settings: SourceProductName=HDL Coder  SourceProductBaseCode=HD
  Bit Shift2 : hdlsllib/Logic and Bit Operations/Bit Shift  mode=Shift Left Logical  N=3
      settings: SourceProductName=HDL Coder  SourceProductBaseCode=HD
  Bit Shift3 : hdlsllib/Logic and Bit Operations/Bit Shift  mode=Shift Right Logical  N=6
      settings: SourceProductName=HDL Coder  SourceProductBaseCode=HD
  Bit Shift4 : hdlsllib/Logic and Bit Operations/Bit Shift  mode=Shift Left Logical  N=1
      settings: SourceProductName=HDL Coder  SourceProductBaseCode=HD
  Bit Shift5 : hdlsllib/Logic and Bit Operations/Bit Shift  mode=Shift Right Logical  N=6
      settings: SourceProductName=HDL Coder  SourceProductBaseCode=HD
  Bit Shift6 : hdlsllib/Logic and Bit Operations/Bit Shift  mode=Shift Right Logical  N=7
      settings: SourceProductName=HDL Coder  SourceProductBaseCode=HD
  Compare To Constant{,5,8,11} (4 alike) : simulink/Logic and Bit Operations/Compare To Constant  relop===  const=0  OutDataTypeStr=boolean
  Compare To Constant{1,6,9,12} (4 alike) : simulink/Logic and Bit Operations/Compare To Constant  relop===  const=1  OutDataTypeStr=boolean
  Compare To Constant10 : simulink/Logic and Bit Operations/Compare To Constant  relop===  const=2  OutDataTypeStr=boolean
  Compare To Constant2 : simulink/Logic and Bit Operations/Compare To Constant  relop===  const=2  OutDataTypeStr=boolean
  Compare To Constant3 : simulink/Logic and Bit Operations/Compare To Constant  relop===  const=3  OutDataTypeStr=boolean
  Compare To Constant4 : simulink/Logic and Bit Operations/Compare To Constant  relop===  const=4  OutDataTypeStr=boolean
  Compare To Constant7 : simulink/Logic and Bit Operations/Compare To Constant  relop===  const=2  OutDataTypeStr=boolean
  Display{1,3..5} (4 alike) : Display
  Mux : Mux  Inputs=5
  Mux1 : Mux  Inputs=3
  Mux2 : Mux  Inputs=3
  Mux3 : Mux  Inputs=2
  Out1 : Outport
  Out2 : Outport  Port=2
  Out3 : Outport  Port=3
  Out4 : Outport  Port=4
  wires:
  In1/1 -> Bit Shift/1, Bit Shift2/1, Bit Shift6/1, Bit Shift4/1
  Bit Shift1/1 -> Compare To Constant/1, Compare To Constant1/1, Compare To Constant2/1, Compare To Constant4/1, Compare To Constant3/1
  Mux/1 -> Out1/1, Display5/1
  Compare To Constant2/1 -> Mux/3
  Compare To Constant4/1 -> Mux/5
  Compare To Constant3/1 -> Mux/4
  Compare To Constant1/1 -> Mux/2  "Licht_AUTO"
  Compare To Constant/1 -> Mux/1
  Bit Shift2/1 -> Bit Shift3/1
  Compare To Constant5/1 -> Mux1/1
  Compare To Constant6/1 -> Mux1/2
  Compare To Constant7/1 -> Mux1/3
  Mux1/1 -> Out2/1, Display1/1
  Bit Shift4/1 -> Bit Shift5/1
  Bit Shift5/1 -> Compare To Constant8/1, Compare To Constant10/1, Compare To Constant9/1
  Compare To Constant8/1 -> Mux2/1
  Compare To Constant10/1 -> Mux2/3
  Compare To Constant9/1 -> Mux2/2
  Compare To Constant12/1 -> Mux3/2
  Compare To Constant11/1 -> Mux3/1
  Bit Shift6/1 -> Compare To Constant11/1, Compare To Constant12/1
  Mux3/1 -> Display4/1, Out4/1
  Bit Shift3/1 -> Compare To Constant7/1, Compare To Constant5/1, Compare To Constant6/1
  Mux2/1 -> Out3/1, Display3/1
  Bit Shift/1 -> Bit Shift1/1

== stateflow chart BlinkerCAN/Steuerung_Licht ==
  state Default
    entry:
    FEL_LED = false
    ABL_LED = false
    TFL_LED = false
  state Automatik_Betrieb
    entry:
    TFL_LED=false
    ABL_LED=false
    FEL_LED=false
  state Hell
    entry:
    TFL_LED=true
    ABL_LED=false
    FEL_LED=false
  state Dunkel
    state Kleiner
      entry:
      TFL_LED=false
      ABL_LED=true
      FEL_LED=false
    state Groesser
      entry:
      TFL_LED=false
      ABL_LED=false
      FEL_LED=true
    (default) -> Groesser
    Kleiner -> Groesser [order 3] : [Distanz > 250]
    Groesser -> Kleiner [order 3] : [Distanz < 250]
    Groesser -> Dunkel [order 1] : [Licht_Auto==0]
    Groesser -> Dunkel [order 2] : [Helligkeit==1]
    Kleiner -> Dunkel [order 2] : [Helligkeit==1]
    Kleiner -> Dunkel [order 1] : [Licht_Auto==0]
  state Tagfahr_Licht
    entry:
    TFL_LED=true
  state Abblend_Licht
    entry:
    ABL_LED=true
  state Fern_Licht
    entry:
    FEL_LED=true
  (default) -> Default
  Automatik_Betrieb -> Hell [order 2] : [Helligkeit==1]
  Default -> Automatik_Betrieb [order 1] : [Licht_Auto==1]
  Automatik_Betrieb -> Default [order 1] : [Licht_Auto==0]
  Hell -> Automatik_Betrieb [order 1] : [Licht_Auto==0]
  Fern_Licht -> Default : [Licht_FEL==0]
  Default -> Fern_Licht [order 2] : [Licht_FEL==1]
  Dunkel -> Hell [order 1] : [Helligkeit==1]
  Hell -> Dunkel [order 2] : [Helligkeit==0]
  Dunkel -> Automatik_Betrieb [order 2] : [Licht_Auto==0]
  Automatik_Betrieb -> Dunkel [order 3] : [Helligkeit==0]
  Default -> Tagfahr_Licht [order 4] : [Licht_TFL==1]
  Tagfahr_Licht -> Default : [Licht_TFL==0]
  Default -> Abblend_Licht [order 3] : [Licht_ABL==1]
  Abblend_Licht -> Default : [Licht_ABL==0]
  data: FEL_LED output; Helligkeit input; Distanz input; ABL_LED output; TFL_LED output; Licht_Auto input; Licht_TFL input; Licht_ABL input; Licht_FEL input

== stateflow chart BlinkerCAN/Steuerung_Blinker ==
  state Dummy
    entry:
    BLL_LED=false;
    BLR_LED=false
    CountL = 1;
    CountR = 1;
    SchliessCount=0;
  state BlinkerR
    entry:
    BLR_LED=true;
  state BlinkerL
    entry:
    BLL_LED=true;
  state BlinkerTipL
    entry:
    BLL_LED=true;
    exit:
    CountL = CountL + 1;
  state EnableBlinkerTipL
    entry:
    BLL_LED = false
  state WarnBlinker
    entry:
    CountL==9;
    CountR==9;
    BLL_LED=true;
    BLR_LED=true;
  state EnableBlinkerTipR
    entry:
    BLR_LED = false
  state BlinkerTipR
    entry:
    BLR_LED=true;
    exit:
    CountR = CountR + 1;
  state SchliessenBlinken1
    entry:
    BLL_LED=true;
    BLR_LED=true;
  state AlarmBlinken
    entry:
    BLL_LED=(~BLL_LED)
    BLR_LED=(~BLR_LED)
  state SchliessenBlinken2
    entry:
    BLL_LED=false;
    BLR_LED=false;
    SchliessCount = SchliessCount + 1;
  state OeffnenBlinken
    entry:
    BLL_LED=true;
    BLR_LED=true;
  (default) -> Dummy
  BlinkerR -> Dummy : after(0.5,sec)
  (junction 223) -> BlinkerR : after(0.5,sec)
  Dummy -> (junction 223) [order 2] : [Blinker_R ==1]
  BlinkerL -> Dummy : after(0.5,sec)
  Dummy -> (junction 221) [order 5] : [Blinker_L ==1]
  (junction 221) -> BlinkerL : after(0.5,sec)
  EnableBlinkerTipL -> Dummy [order 1] : [Warnblinker == 1 || CountL > 3 || Blinker_R == 1 || Blinker_Tip_R == 1]
  EnableBlinkerTipL -> (junction 225) [order 2] : [CountL <= 3]
  (junction 225) -> BlinkerTipL : after(0.5,sec)
  BlinkerTipL -> EnableBlinkerTipL : after(0.5,sec)
  Dummy -> EnableBlinkerTipL [order 6] : [Blinker_Tip_L == 1 && Warnblinker == 0]
  EnableBlinkerTipR -> (junction 227) [order 2] : [CountR <= 3]
  (junction 227) -> BlinkerTipR : after(0.5,sec)
  (junction 230) -> WarnBlinker : after(0.5,sec)
  Dummy -> (junction 230) [order 1] : [Warnblinker==1]
  EnableBlinkerTipR -> Dummy [order 1] : [Warnblinker == 1 || CountR > 3 || Blinker_L == 1 || Blinker_Tip_L == 1]
  BlinkerTipR -> EnableBlinkerTipR : after(0.5,sec)
  Dummy -> EnableBlinkerTipR [order 7] : [Blinker_Tip_R == 1 && Warnblinker == 0]
  WarnBlinker -> Dummy : after(0.5,sec)
  AlarmBlinken -> Dummy [order 1] : [AlarmZustand==0]
  Dummy -> AlarmBlinken [order 3] : [AlarmZustand==1]
  Dummy -> OeffnenBlinken [order 8] : [SchliessZustand==0 && Trigger_SchliessZustand==1]
  OeffnenBlinken -> Dummy : after(0.5,sec)
  Dummy -> SchliessenBlinken1 [order 4] : [SchliessZustand == 1 && Trigger_SchliessZustand==1]
  (junction 244) -> Dummy : after(0.5,sec)
  SchliessenBlinken1 -> (junction 244) [order 1] : [SchliessCount == 1]
  SchliessenBlinken2 -> SchliessenBlinken1 : after(0.5,sec)
  SchliessenBlinken1 -> (junction 247) [order 2] : [SchliessCount<1]
  (junction 247) -> SchliessenBlinken2 : after(0.5,sec)
  AlarmBlinken -> AlarmBlinken [order 2] : after(1,sec)
  data: BLL_LED output boolean; BLR_LED output boolean; Blinker_Tip_R input; Blinker_R input; Blinker_Tip_L input; Blinker_L input; Warnblinker input; SchliessZustand input; AlarmZustand input; CountL local double [0..10] =9; OpeningCount local; ClosingCount local; Opening local; Closing local; Blinkertip local =0; CountR local =9; Trigger_SchliessZustand input; SchliessCount local
